simulink model "bh_CONCEPT_scope_layout_check"  (R2015b)
settings: Solver=ode45  StartTime=0.0  StopTime=10  FixedStep=0.001  RelTol=1e-3
settings Model: Creator=bhorton  LastModifiedBy=bhorton
settings DataIOCC: LimitDataPoints=off  SaveOutput=off  SignalLogging=off  DSMLogging=off  VisualizeSimOutput=off  SaveTime=off

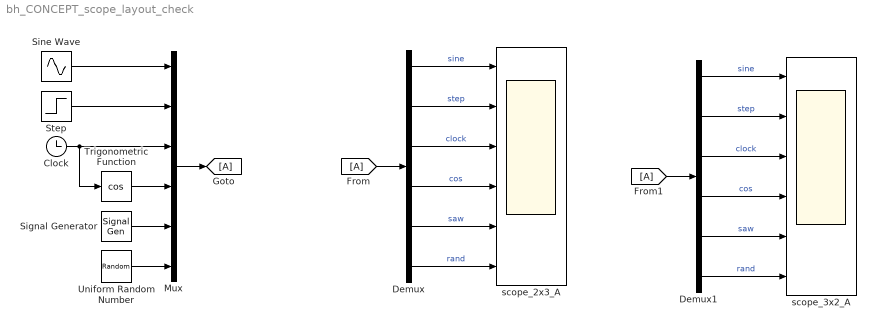
== system bh_CONCEPT_scope_layout_check ==
  Clock : Clock
  Demux : Demux  Outputs=6
  Demux1 : Demux  Outputs=6
  Mux : Mux  Inputs=6
  Signal Generator : SignalGenerator  WaveForm=sawtooth  Frequency=0.5
  Sine Wave : Sin  SampleTime=0
  Step : Step  SampleTime=0
  Trigonometric Function : Trigonometry  Operator=cos
  Uniform Random Number : UniformRandomNumber  SampleTime=0.1
  scope_2x3_A : Scope  NumInputPorts=6
  scope_3x2_A : Scope  NumInputPorts=6
  wires:
  Step/1 -> Mux/2
  Sine Wave/1 -> Mux/1
  Clock/1 -> Trigonometric Function/1, Mux/3
  Trigonometric Function/1 -> Mux/4
  Signal Generator/1 -> Mux/5
  Uniform Random Number/1 -> Mux/6
  Mux/1 -> [A]
  [A] -> Demux/1
  Demux/6 -> scope_2x3_A/6  "rand"
  Demux/5 -> scope_2x3_A/5  "saw"
  Demux/4 -> scope_2x3_A/4  "cos"
  Demux/3 -> scope_2x3_A/3  "clock"
  Demux/2 -> scope_2x3_A/2  "step"
  Demux/1 -> scope_2x3_A/1  "sine"
  [A] -> Demux1/1
  Demux1/6 -> scope_3x2_A/6  "rand"
  Demux1/5 -> scope_3x2_A/5  "saw"
  Demux1/4 -> scope_3x2_A/4  "cos"
  Demux1/3 -> scope_3x2_A/3  "clock"
  Demux1/2 -> scope_3x2_A/2  "step"
  Demux1/1 -> scope_3x2_A/1  "sine"
